simulink model "Nezavisimoe"  (R2022a)
settings: Solver=ode23tb  StartTime=0.0  StopTime=inf  MaxStep=1e-3  RelTol=1e-3
undefined symbols (not defined in the file): CF, Es, Imax, lamda, RaLa, ReLe, Rsh0, step, Tokivx, Udnom, Udnom1, Vmax, Vnach
libraries: spsControlledVoltageSourceLib x4, spsSeriesRLCBranchLib x3, spsCurrentMeasurementLib x2, simulink x1, spsDiodeLib x1, spspowerguiLib x1
settings Model: PacingRate=1000  Creator=админ  LastModifiedBy=админ
settings SolverCC: ZeroCrossAlgorithm=Adaptive
settings DebuggingCC: IgnoredZcDiagnostic=none

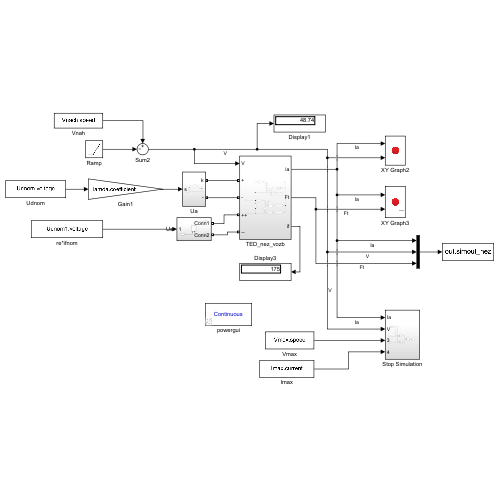
[thumbnail: Simulink's stored preview of the top-level diagram]
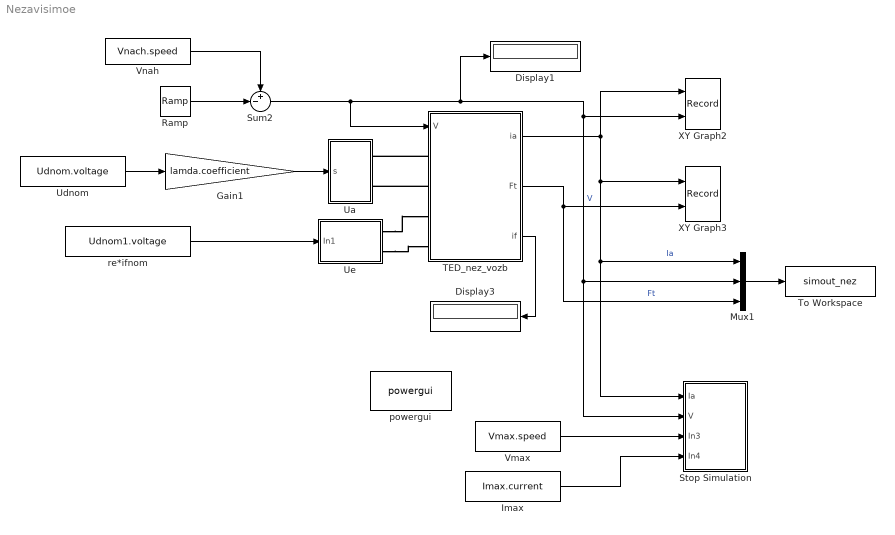
== system Nezavisimoe ==
  Display1 : Display
  Display3 : Display
  Gain1 : Gain  Gain=lamda.coefficient
  Imax : Constant  Value=Imax.current
  Mux1 : Mux  Inputs=3
  Ramp : simulink/Sources/Ramp  slope=0.2  start=0  InitialOutput=0
  Stop Simulation : Subsystem
  Sum2 : Sum  Inputs=+-|
  TED_nez_vozb : Subsystem
  To Workspace : ToWorkspace  VariableName=simout_nez  SaveFormat=Structure  SampleTime=step.measurementsnez
      settings: Save2DSignal=2-D array (concatenate along first dimension)
  Ua : Subsystem
  Udnom : Constant  Value=Udnom.voltage
  Ue : Subsystem
  Vmax : Constant  Value=Vmax.speed
  Vnah : Constant  Value=Vnach.speed
  XY Graph2 : Record  FileSettingsInternal="{\"entries\":[{\"content\":{\"excelSettings\":{\"content\":{},\"type\":\"Streamout.ExcelSettings\"}},\"type\":\"Streamout.FileSettingStorage\",\"uuid\":\"f89055a0-f198-4fb3-a9c9-daac39fdd426\"}],\"packageUris\":[\"http://schema.mathworks.com/mf0/streamout_blocks/R2020a\"],\"version\":\"1.0\"}"  Layout=[1 1]  SignalsInternal="{\"entries\":[{\"content\":{\"signals\":[{\"content\":{\"blockPath\":[\"Nezavisimoe/XY Graph2\"],\"channel\":[],\"dimensions\":[1],\"domain\":\"Nezavisimoe/XY Graph2\",\"lineColor\":\"#a2142f\",\"plots\":[1],\"port\":1,\"sid\":[\"\"],\"signalID\":141881,\"signalName\":\"Ia\"},\"type\":\"RecordBlkView.Signal\",\"uuid\":\"5273f552-5626-43fe-9697-ea22cb94ba72\"},{\"content\":{\"blockPath\":[\"Nezavisimoe/XY Graph2\"],\"channel\":[],\"dimensions\":[1],\"domain\":\"Nezavisimoe/XY Graph2\",\"lineColor\":\"#139fff\",\"plots\":[1],\"port\":2,\"sid\":[\"\"],\"signalID\":141885,\"signalName\":\"V\"},\"type\":\"RecordBlkView.Signal\",\"uuid\":\"39397d46-fd33-4fc4-a743-033059d517d8\"}]},\"type\":\"RecordBlkView.InputSignals\",\"uuid\":\"df61917a-6342-4aeb-b0bd-c365c2b03ad8\"}],\"packageUris\":[\"http://schema.mathworks.com/mf0/streamout_blocks/R2020a\"],\"version\":\"1.0\"}"  VisualizationBindings="{\"xyplotplugin\":{\"info\":[{\"series\":[{\"bindingParametersList\":[{\"parameter\":\"X-Axis\",\"signalID\":141881,\"signalName\":\"Ia\"},{\"parameter\":\"Y-Axis\",\"signalID\":141885,\"signalName\":\"V\"}],\"seriesID\":8215}],\"subplotID\":1}]}}"  CompatibilityTag=XY  st=-1
  XY Graph3 : Record  FileSettingsInternal="{\"entries\":[{\"content\":{\"excelSettings\":{\"content\":{},\"type\":\"Streamout.ExcelSettings\"}},\"type\":\"Streamout.FileSettingStorage\",\"uuid\":\"c9ebc919-2905-41f4-8dbe-0dc1d3685c32\"}],\"packageUris\":[\"http://schema.mathworks.com/mf0/streamout_blocks/R2020a\"],\"version\":\"1.0\"}"  Layout=[1 1]  SignalsInternal="{\"entries\":[{\"content\":{\"signals\":[{\"content\":{\"blockPath\":[\"Nezavisimoe/XY Graph3\"],\"channel\":[],\"dimensions\":[1],\"domain\":\"Nezavisimoe/XY Graph3\",\"lineColor\":\"#a2142f\",\"plots\":[1],\"port\":1,\"sid\":[\"\"],\"signalID\":141889,\"signalName\":\"Ia\"},\"type\":\"RecordBlkView.Signal\",\"uuid\":\"49625309-aa73-4531-8b7f-4180b13e841e\"},{\"content\":{\"blockPath\":[\"Nezavisimoe/XY Graph3\"],\"channel\":[],\"dimensions\":[1],\"domain\":\"Nezavisimoe/XY Graph3\",\"lineColor\":\"#139fff\",\"plots\":[1],\"port\":2,\"sid\":[\"\"],\"signalID\":141893,\"signalName\":\"Ft\"},\"type\":\"RecordBlkView.Signal\",\"uuid\":\"ddd44c21-6f1d-4705-9ce1-1f751ad22ba5\"}]},\"type\":\"RecordBlkView.InputSignals\",\"uuid\":\"ae23293b-bf4d-4116-bc3a-f236d6890bc5\"}],\"packageUris\":[\"http://schema.mathworks.com/mf0/streamout_blocks/R2020a\"],\"version\":\"1.0\"}"  VisualizationBindings="{\"xyplotplugin\":{\"info\":[{\"series\":[{\"bindingParametersList\":[{\"parameter\":\"X-Axis\",\"signalID\":141889,\"signalName\":\"Ia\"},{\"parameter\":\"Y-Axis\",\"signalID\":141893,\"signalName\":\"Ft\"}],\"seriesID\":21470}],\"subplotID\":1}]}}"  CompatibilityTag=XY  st=-1
  powergui : spspowerguiLib/powergui  Priority=1  SimulationMode=Continuous  SampleTime=50e-6  frequency=60  Iterations=50  frequencyindice=0  Pbase=100e6  ErrMax=1e-4  UnitsV=kV  UnitsW=MW  buscounter=0  FunctionMessages=off  echomessages=off  EnableUseOfTLC=off  CurrentSourceSwitches=off  DisableSnubberDevices=off  DisableRonSwitches=off  DisableVfSwitches=off  DisplayEquations=off  AutomaticDiscreteSolvers=off  SolverType=Tustin/Backward Euler (TBE)  Interpol=off  ExternalGateDelay=off  methode=off  Ts=100  x0status=blocks  SPID=on  SwTol=0  HookPort=off  NonlinearTolerance=1e-4  nMaxIteration=100  ContinueOnMaxIteration=off  RestoreLinks=warning  ResistiveCurrentMeasurement=off  Frange=[0:2:500]  Ylog=off  Xlog=on  ShowGrid=off  save=off  variable=ZData  structure=0  ZoomFFT=off  StartTime=0.0  cycles=1  DisplayStyle=1  fundamental=60  FreqAxis=off  MaxFrequency=1000  frequencyindicesteady=1  RmsSteady=1  display=off
  re*ifnom : Constant  Value=Udnom1.voltage
  wires:
  Udnom/1 -> Gain1/1
  Gain1/1 -> Ua/1(s)
  re*ifnom/1 -> Ue/1(In1)
  Ramp/1 -> Sum2/2
  Vnah/1 -> Sum2/1
  Sum2/1 -> TED_nez_vozb/1(V), Stop Simulation/2(V), Mux1/2, XY Graph2/2, Display1/1  "V"
  TED_nez_vozb/1(ia) -> XY Graph3/1, Stop Simulation/1(Ia), Mux1/1, XY Graph2/1  "Ia"
  TED_nez_vozb/2(Ft) -> Mux1/3, XY Graph3/2  "Ft"
  TED_nez_vozb/3(if) -> Display3/1
  Vmax/1 -> Stop Simulation/3(In3)
  Imax/1 -> Stop Simulation/4(In4)
  Mux1/1 -> To Workspace/1
  connections:
  TED_nez_vozb/LConn1 -- Ua/RConn1
  TED_nez_vozb/LConn2 -- Ua/RConn2
  Ue/RConn2 -- TED_nez_vozb/LConn4
  Ue/RConn1 -- TED_nez_vozb/LConn3

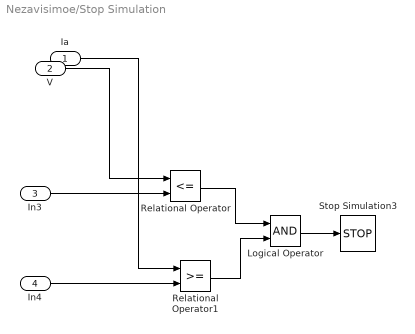
== system Nezavisimoe/Stop Simulation ==
  Ia : Inport
  V : Inport  Port=2
  In3 : Inport  Port=3
  In4 : Inport  Port=4
  Logical Operator : Logic  AllPortsSameDT=off  OutDataTypeStr=boolean
  Relational Operator : RelationalOperator  Operator=<=  OutDataTypeStr=boolean  RndMeth=Simplest  InputSameDT=off
  Relational Operator1 : RelationalOperator  OutDataTypeStr=boolean  RndMeth=Simplest  InputSameDT=off
  Stop Simulation3 : Stop
  wires:
  Ia/1 -> Relational Operator1/1
  Logical Operator/1 -> Stop Simulation3/1
  V/1 -> Relational Operator/1
  Relational Operator/1 -> Logical Operator/1
  Relational Operator1/1 -> Logical Operator/2
  In3/1 -> Relational Operator/2
  In4/1 -> Relational Operator1/2

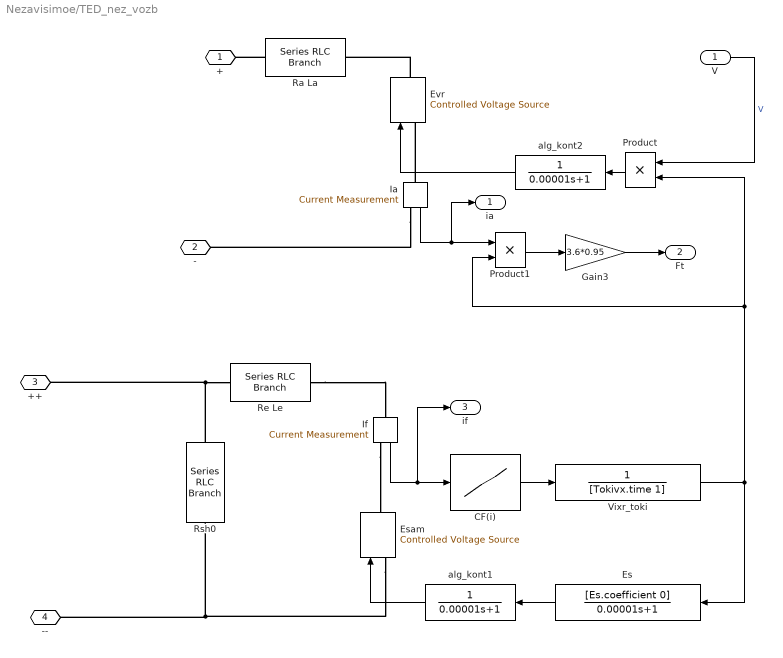
== system Nezavisimoe/TED_nez_vozb ==
  V : Inport
  CF(i) : Lookup_n-D  NumberOfTableDimensions=1  BreakpointsForDimension1=CF.currentvozb  Table=CF.CvF  InternalRulePriority=Speed  RndMeth=Simplest
  Es : TransferFcn  Numerator=[Es.coefficient 0]  Denominator=[0.00001 1]
  Esam : spsControlledVoltageSourceLib/Controlled Voltage Source  Initialize=on  Source_Type=AC  Amplitude=0  Phase=0  Frequency=0  Measurements=None
  Evr : spsControlledVoltageSourceLib/Controlled Voltage Source  Initialize=on  Source_Type=AC  Amplitude=0  Phase=0  Frequency=0  Measurements=None
  Gain3 : Gain  Gain=3.6*0.95
  Ia : spsCurrentMeasurementLib/Current Measurement  PhasorSimulation=off  OutputType=Complex  PSBequivalent=0
  If : spsCurrentMeasurementLib/Current Measurement  PhasorSimulation=off  OutputType=Complex  PSBequivalent=0
  Product : Product
  Product1 : Product
  Ra La : spsSeriesRLCBranchLib/Series RLC Branch  LConnTagsString=__new0  RConnTagsString=__new0  BranchType=RL  Resistance=RaLa.Res  Inductance=RaLa.Ind  SetiL0=off  InitialCurrent=0  Capacitance=1e-6  Setx0=off  InitialVoltage=0  Measurements=None
  Re Le : spsSeriesRLCBranchLib/Series RLC Branch  LConnTagsString=__new0  RConnTagsString=__new0  BranchType=RL  Resistance=ReLe.Res  Inductance=ReLe.Ind  SetiL0=off  InitialCurrent=0  Capacitance=1e-6  Setx0=off  InitialVoltage=0  Measurements=None
  Rsh0 : spsSeriesRLCBranchLib/Series RLC Branch  LConnTagsString=__new0  RConnTagsString=__new0  BranchType=R  Resistance=Rsh0.Res  Inductance=1e-3  SetiL0=off  InitialCurrent=0  Capacitance=1e-6  Setx0=off  InitialVoltage=0  Measurements=None
  Vixr_toki : TransferFcn  Denominator=[Tokivx.time 1]
  alg_kont1 : TransferFcn  Denominator=[0.00001 1]
  alg_kont2 : TransferFcn  Denominator=[0.00001 1]
  + : PMIOPort  Side=Left
  - : PMIOPort  Port=2  Side=Left
  ++ : PMIOPort  Port=3  Side=Left
  -- : PMIOPort  Port=4  Side=Left
  ia : Outport
  Ft : Outport  Port=2
  if : Outport  Port=3
  wires:
  alg_kont2/1 -> Evr/1
  Vixr_toki/1 -> Product1/2, Product/2, Es/1
  Ia/1 -> ia/1, Product1/1
  Product1/1 -> Gain3/1
  Product/1 -> alg_kont2/1
  Es/1 -> alg_kont1/1
  If/1 -> if/1, CF(i)/1
  alg_kont1/1 -> Esam/1
  CF(i)/1 -> Vixr_toki/1
  V/1 -> Product/1  "V"
  Gain3/1 -> Ft/1
  connections:
  Ia/LConn1 -- Evr/LConn1
  Evr/RConn1 -- Ra La/RConn1
  Rsh0/LConn1 -- ++/RConn1 -- Re Le/LConn1
  If/RConn1 -- Esam/RConn1
  Ia/RConn1 -- -/RConn1
  Esam/LConn1 -- --/RConn1 -- Rsh0/RConn1
  Re Le/RConn1 -- If/LConn1
  Ra La/LConn1 -- +/RConn1

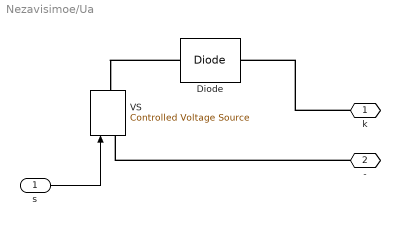
== system Nezavisimoe/Ua ==
  s : Inport
  Diode : spsDiodeLib/Diode  Ron=0.001  Lon=0  Vf=0.8  IC=0  UseSnubber=0  Rs=500  Cs=250e-9  Measurements=off
  VS : spsControlledVoltageSourceLib/Controlled Voltage Source  Initialize=on  Source_Type=AC  Amplitude=0  Phase=0  Frequency=0  Measurements=None
  k : PMIOPort  Side=Right
  - : PMIOPort  Port=2  Side=Right
  wires:
  s/1 -> VS/1
  connections:
  Diode/LConn1 -- VS/RConn1
  k/RConn1 -- Diode/RConn1
  -/RConn1 -- VS/LConn1

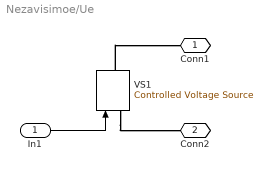
== system Nezavisimoe/Ue ==
  In1 : Inport
  VS1 : spsControlledVoltageSourceLib/Controlled Voltage Source  Initialize=on  Source_Type=AC  Amplitude=0  Phase=0  Frequency=0  Measurements=None
  Conn1 : PMIOPort  Side=Right
  Conn2 : PMIOPort  Port=2  Side=Right
  wires:
  In1/1 -> VS1/1
  connections:
  VS1/LConn1 -- Conn2/RConn1
  VS1/RConn1 -- Conn1/RConn1
